simulink model "Examen2"  (R2013a)
settings: Solver=ode23  StartTime=0.0  StopTime=10.0  RelTol=1e-3
libraries: powerlib x23, powerlib_meascontrol x4
settings Model: Creator=Miguel  LastModifiedBy=Miguel

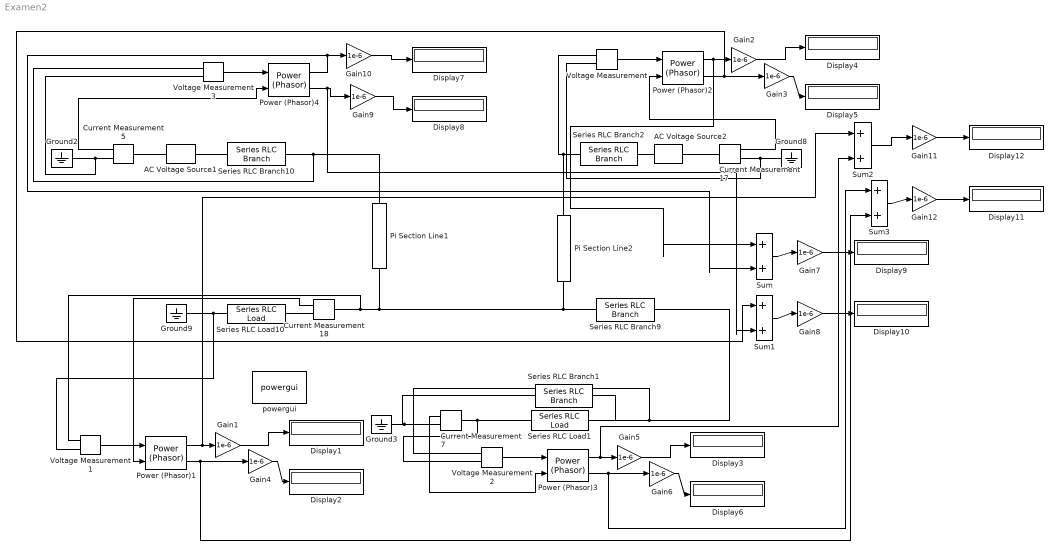
== system Examen2 ==
  AC Voltage Source1 : powerlib/Electrical Sources/AC Voltage Source  Amplitude=1.0*100e3*sqrt(2)  Phase=0  Frequency=60  SampleTime=0  Measurements=None
  AC Voltage Source2 : powerlib/Electrical Sources/AC Voltage Source  Amplitude=0.9800*100e3*sqrt(2)  Phase=0.0712  Frequency=60  SampleTime=0  Measurements=None
  Current Measurement{5,7,17..18} (4 alike) : powerlib/Measurements/Current Measurement  PhasorSimulation=on  OutputType=Complex  PSBequivalent=0
  Display{1..12} (12 alike) : Display
  Gain{1..12} (12 alike) : Gain  Gain=1e-6
  Ground{2..3,8..9} (4 alike) : powerlib/Elements/Ground  LConnTagsString=a
  Pi Section Line1 : powerlib/Elements/Pi Section Line  LConnTagsString=__new0  RConnTagsString=__new0  Frequency=60  Resistance=0.001*100e3^2/100e6  Inductance=0.05/(2*pi*60)*100e3^2/100e6  Capacitance=0.1/(2*pi*60*100e3^2/100e6)  Length=1  PiSections=1  Measurements=None
      settings: AttributesFormatString=\n
  Pi Section Line2 : powerlib/Elements/Pi Section Line  LConnTagsString=__new0  RConnTagsString=__new0  Frequency=60  Resistance=0.001*100e3^2/100e6  Inductance=0.05/(2*pi*60)*100e3^2/100e6  Capacitance=0.1/(2*pi*60*100e3^2/100e6)  Length=1  PiSections=1  Measurements=None
      settings: AttributesFormatString=\n
  Power (Phasor){1..4} (4 alike) : powerlib_meascontrol/Measurements/Power (Phasor)
  Series RLC Branch1 : powerlib/Elements/Series RLC Branch  LConnTagsString=__new0  RConnTagsString=__new0  BranchType=C  Resistance=0  Inductance=0.1/(2*pi*60)*100e3^2/100e6  SetiL0=off  InitialCurrent=0  Capacitance=0.1/(2*pi*60*100e3^2/100e6)  Setx0=off  InitialVoltage=0  Measurements=None
  Series RLC Branch10 : powerlib/Elements/Series RLC Branch  LConnTagsString=__new0  RConnTagsString=__new0  BranchType=R  Resistance=1e-5  Inductance=1e-3  SetiL0=off  InitialCurrent=0  Capacitance=1e-6  Setx0=off  InitialVoltage=0  Measurements=None
  Series RLC Branch2 : powerlib/Elements/Series RLC Branch  LConnTagsString=__new0  RConnTagsString=__new0  BranchType=R  Resistance=1e-5  Inductance=1e-3  SetiL0=off  InitialCurrent=0  Capacitance=1e-6  Setx0=off  InitialVoltage=0  Measurements=None
  Series RLC Branch9 : powerlib/Elements/Series RLC Branch  LConnTagsString=__new0  RConnTagsString=__new0  BranchType=L  Resistance=0  Inductance=0.1/(2*pi*60)*100e3^2/100e6  SetiL0=off  InitialCurrent=0  Capacitance=1e-6  Setx0=off  InitialVoltage=0  Measurements=None
  Series RLC Load1 : powerlib/Elements/Series RLC Load  LConnTagsString=a  RConnTagsString=__new0  NominalVoltage=0.6922*100e3  NominalFrequency=60  ActivePower=100e6  InductivePower=100e6  CapacitivePower=0  Setx0=off  InitialVoltage=0  SetiL0=off  InitialCurrent=0  Measurements=Branch current
  Series RLC Load10 : powerlib/Elements/Series RLC Load  LConnTagsString=a  RConnTagsString=__new0  NominalVoltage=0.9264*100e3  NominalFrequency=60  ActivePower=100e6  InductivePower=100e6  CapacitivePower=0  Setx0=off  InitialVoltage=0  SetiL0=off  InitialCurrent=0  Measurements=Branch current
  Sum{,1..3} (4 alike) : Sum  Inputs=|++
  Voltage Measurement{,1..3} (4 alike) : powerlib/Measurements/Voltage Measurement  PhasorSimulation=on  OutputType=Complex  PSBequivalent=0
  powergui : powerlib/powergui  Priority=1  SimulationMode=Phasor  SolverType=Tustin  SampleTime=50e-6  frequency=60  SPID=off  DisableSnubberDevices=off  DisableRonSwitches=off  DisableVfSwitches=off  SwTol=0  Interpol=off  DisplayEquations=off  frequencyindice=60  Pbase=100e6  ErrMax=1e-4  Iterations=50  UnitsV=kV  UnitsW=MW  FunctionMessages=off  echomessages=off  HookPort=off  EnableUseOfTLC=off  x0status=blocks  RestoreLinks=warning  ResistiveCurrentMeasurement=off  Frange=[0:2:500]  Ylog=off  Xlog=on  ShowGrid=off  save=off  variable=ZData  ZoomFFT=off  StartTime=0.0  cycles=1  DisplayStyle=1  fundamental=60  FreqAxis=off  MaxFrequency=1000  frequencyindicesteady=1  RmsSteady=2  display=off  Ts=0  methode=off
  wires:
  Power (Phasor)2/1 -> Sum/1, Gain2/1
  Power (Phasor)2/2 -> Sum1/1, Gain3/1
  Gain2/1 -> Display4/1
  Gain3/1 -> Display5/1
  Voltage Measurement/1 -> Power (Phasor)2/1
  Current Measurement17/1 -> Power (Phasor)2/2
  Power (Phasor)1/1 -> Sum2/1, Gain1/1
  Power (Phasor)1/2 -> Sum3/2, Gain4/1
  Gain1/1 -> Display1/1
  Gain4/1 -> Display2/1
  Voltage Measurement1/1 -> Power (Phasor)1/1
  Current Measurement18/1 -> Power (Phasor)1/2
  Power (Phasor)3/1 -> Sum2/2, Gain5/1
  Gain5/1 -> Display3/1
  Gain6/1 -> Display6/1
  Voltage Measurement2/1 -> Power (Phasor)3/1
  Current Measurement7/1 -> Power (Phasor)3/2
  Voltage Measurement3/1 -> Power (Phasor)4/1
  Current Measurement5/1 -> Power (Phasor)4/2
  Gain9/1 -> Display8/1
  Power (Phasor)4/1 -> Gain10/1, Sum/2
  Gain10/1 -> Display7/1
  Sum/1 -> Gain7/1
  Gain7/1 -> Display9/1
  Sum1/1 -> Gain8/1
  Gain8/1 -> Display10/1
  Sum2/1 -> Gain11/1
  Gain11/1 -> Display12/1
  Sum3/1 -> Gain12/1
  Gain12/1 -> Display11/1
  Power (Phasor)4/2 -> Sum1/2, Gain9/1
  Power (Phasor)3/2 -> Sum3/1, Gain6/1
  connections:
  Series RLC Branch9/LConn1 -- Pi Section Line2/RConn1 -- Pi Section Line1/RConn1 -- Voltage Measurement1/LConn1 -- Current Measurement18/LConn1
  Series RLC Branch10/RConn1 -- Voltage Measurement3/LConn1 -- Pi Section Line1/LConn1
  Pi Section Line2/LConn1 -- Voltage Measurement/LConn1 -- Series RLC Branch2/RConn1
  Current Measurement5/RConn1 -- Voltage Measurement3/LConn2 -- Ground2/LConn1
  Series RLC Branch10/LConn1 -- AC Voltage Source1/RConn1
  Current Measurement5/LConn1 -- AC Voltage Source1/LConn1
  Current Measurement7/RConn1 -- Series RLC Branch1/RConn1 -- Ground3/LConn1
  Voltage Measurement2/LConn2 -- Series RLC Load1/RConn1 -- Current Measurement7/LConn1
  Voltage Measurement2/LConn1 -- Series RLC Branch1/LConn1 -- Series RLC Load1/LConn1 -- Series RLC Branch9/RConn1
  Current Measurement17/RConn1 -- Voltage Measurement/LConn2 -- Ground8/LConn1
  Series RLC Load10/LConn1 -- Voltage Measurement1/LConn2 -- Ground9/LConn1
  Current Measurement18/RConn1 -- Series RLC Load10/RConn1
  AC Voltage Source2/LConn1 -- Current Measurement17/LConn1
  Series RLC Branch2/LConn1 -- AC Voltage Source2/RConn1
